simulink model "MotorSim1"  (R2023b)
settings: Solver=VariableStepAuto  StartTime=0.0  StopTime=10.0  FixedStep=0.001  RelTol=1e-3
undefined symbols (not defined in the file or in its folder): P_tf_d, P_tf_n, V_tf_d, V_tf_n
settings Model: Creator=Joe  LastModifiedBy=root
settings ModelReferenceCC: EnableRefExpFcnMdlSchedulingChecks=on

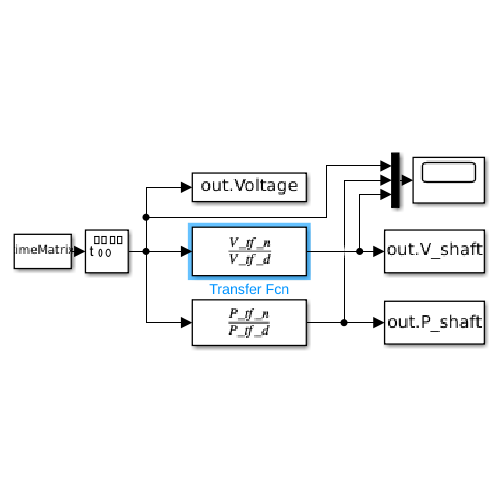
[thumbnail: Simulink's stored preview of the top-level diagram]
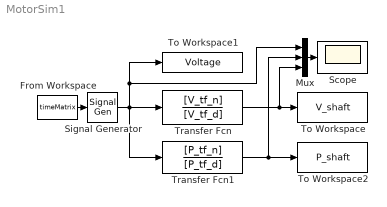
== system MotorSim1 ==
  From Workspace : FromWorkspace  VariableName=timeMatrix
  Mux : Mux  Inputs=3
  Scope : Scope
  Signal Generator : SignalGenerator  WaveForm=square  TimeSource=Use external signal  Amplitude=2  Frequency=0.4
  To Workspace : ToWorkspace  VariableName=V_shaft  SaveFormat=Timeseries  SampleTime=-1
  To Workspace1 : ToWorkspace  VariableName=Voltage  SaveFormat=Timeseries  SampleTime=-1
  To Workspace2 : ToWorkspace  VariableName=P_shaft  SaveFormat=Timeseries  SampleTime=-1
  Transfer Fcn : TransferFcn  Numerator=[V_tf_n]  Denominator=[V_tf_d]
  Transfer Fcn1 : TransferFcn  Numerator=[P_tf_n]  Denominator=[P_tf_d]
  wires:
  Transfer Fcn/1 -> Mux/3, To Workspace/1
  Mux/1 -> Scope/1
  Transfer Fcn1/1 -> Mux/2, To Workspace2/1
  Signal Generator/1 -> Transfer Fcn1/1, Transfer Fcn/1, To Workspace1/1, Mux/1
  From Workspace/1 -> Signal Generator/1
